simulink library "TLCLib"  (R2016b)
settings: Solver=VariableStepAuto  StartTime=0.0  StopTime=10.0  RelTol=1e-3
undefined symbols (not defined in the file): SC_TrqMax_P
libraries: simulink x1
settings Model: Creator=Administrator  LastModifiedBy=Administrator

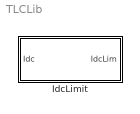
== system TLCLib ==
  IdcLimit : Subsystem  TreatAsAtomicUnit=on

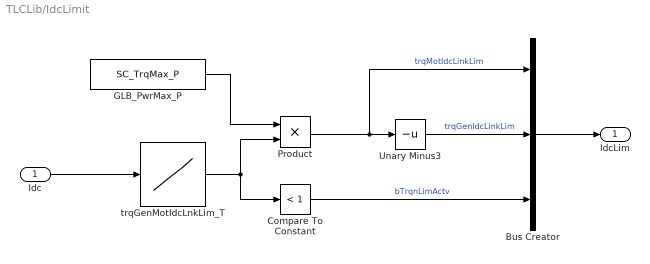
== system TLCLib/IdcLimit ==
  "Idc " : Inport
  Bus Creator : BusCreator  Inputs=3
  Compare To Constant : simulink/Logic and Bit Operations/Compare To Constant  relop=<  const=1  OutDataTypeStr=boolean
  GLB_PwrMax_P : Constant  Value=SC_TrqMax_P  OutDataTypeStr=single
      mask Display:
      | tmpx = get_param(gcbh,'Value');
      | a= evalin('base',[tmpx,'.Value;']);
      | disp([tmpx,': ',num2str(a)]);
  Product : Product
  Unary Minus3 : UnaryMinus
  trqGenMotIdcLnkLim_T : Lookup_n-D  NumberOfTableDimensions=1  DataSpecification=Lookup table object  LookupTableObject=trqGenMotIdcLnkLim_T  BreakpointsForDimension1=[-3500 -3000 0 7000 7200]  BeginIndexSearchUsingPreviousIndexResult=on  Table=[0 1 1 1 0]  ExtrapMethod=Clip  UseLastTableValue=on  InternalRulePriority=Speed  RndMeth=Simplest  InputSameDT=on
  IdcLim : Outport
  wires:
  "Idc "/1 -> trqGenMotIdcLnkLim_T/1
  Unary Minus3/1 -> Bus Creator/2  "trqGenIdcLinkLim"
  trqGenMotIdcLnkLim_T/1 -> Compare To Constant/1, Product/2
  Compare To Constant/1 -> Bus Creator/3  "bTrqnLimActv"
  Bus Creator/1 -> IdcLim/1
  GLB_PwrMax_P/1 -> Product/1
  Product/1 -> Bus Creator/1, Unary Minus3/1  "trqMotIdcLinkLim"
